simulink model "motoman_enghouse"  (Simulink 6.2)
settings: Solver=ode45  SolverMode=SingleTasking  StartTime=0.0  StopTime=10.0  RelTol=1e-3  AbsTol=1e-6
settings Model: Creator=The MathWorks Inc.  LastModifiedBy=Administrator  ExtModeTrigMode=oneshot  ExtModeArmWhenConnect=off  ExtModeAutoUpdateStatusClock=off
settings DataIOCC: LimitDataPoints=off  SignalLoggingName=logsOut
settings OptimizationCC: BooleanDataType=off  InlineInvariantSignals=on
settings DebuggingCC: CheckExecutionContextPreStartOutputMsg=on  CheckExecutionContextRuntimeOutputMsg=on  IntegerOverflowMsg=none
settings HardwareCC: TargetUnknown=on
settings ModelReferenceCC: UpdateModelReferenceTargets=IfOutOfDate

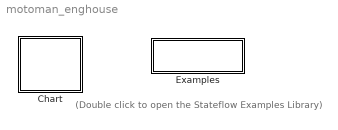
== system motoman_enghouse ==
  note: (Double click to open the
      | Stateflow Examples Library)
  Chart : Stateflow chart
  Examples : Subsystem
      settings: OpenFcn=sf('Private','sf_examples')
      mask Display: disp('Examples')

== system motoman_enghouse/Examples ==

== stateflow chart Chart ==
  state Initialize
    Aquateen\HP3JC\HP3JC.connect_Initialize()
    Aquateen\HP3JC\HP3JC.servo_ServoOn()
    Aquateen\HP3JC\HP3JC.servo_ServoOn()
    Aquateen\HP3JC\HP3JC.error_ClearAlarm()
    Aquateen\HP3JC\StateMachine.Wait(500)
  state RunJob
    Aquateen\HP3JC\HP3JC.job_CopyTextQueue()
    Aquateen\HP3JC\HP3JC.job_SelectJob()
    Aquateen\HP3JC\HP3JC.job_StartJob()
    Aquateen\HP3JC\StateMachine.Wait(8000)
  state Stop
    Aquateen\HP3JC\HP3JC.connect_Disconnect()
  state RunJob2
    Aquateen\HP3JC\HP3JC.job_StartJob()
    Aquateen\HP3JC\StateMachine.Wait(8000)
  state RunJob3
    Aquateen\HP3JC\HP3JC.job_StartJob()
    Aquateen\HP3JC\StateMachine.Wait(8000)
  (default) -> Initialize : Start
  RunJob3 -> Stop : Signal="Stop"
  Initialize -> RunJob : Default
  RunJob -> RunJob2 : Default
  RunJob2 -> RunJob3 : Default
